simulink model "LukePractice"  (R2025a)
settings: Solver=VariableStepAuto  StartTime=0.0  StopTime=10.0  RelTol=1e-3
settings Model: Creator=jakeo  LastModifiedBy=lukef

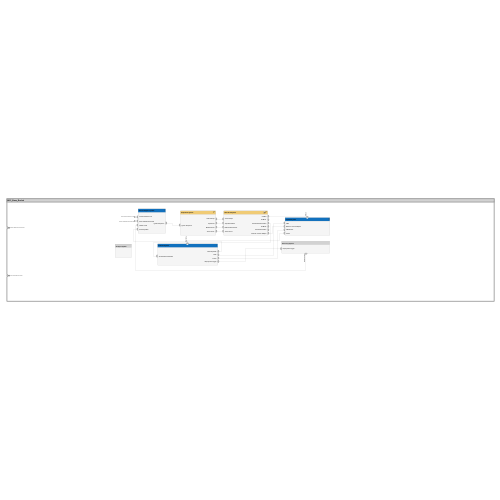
[thumbnail: Simulink's stored preview of the top-level diagram]
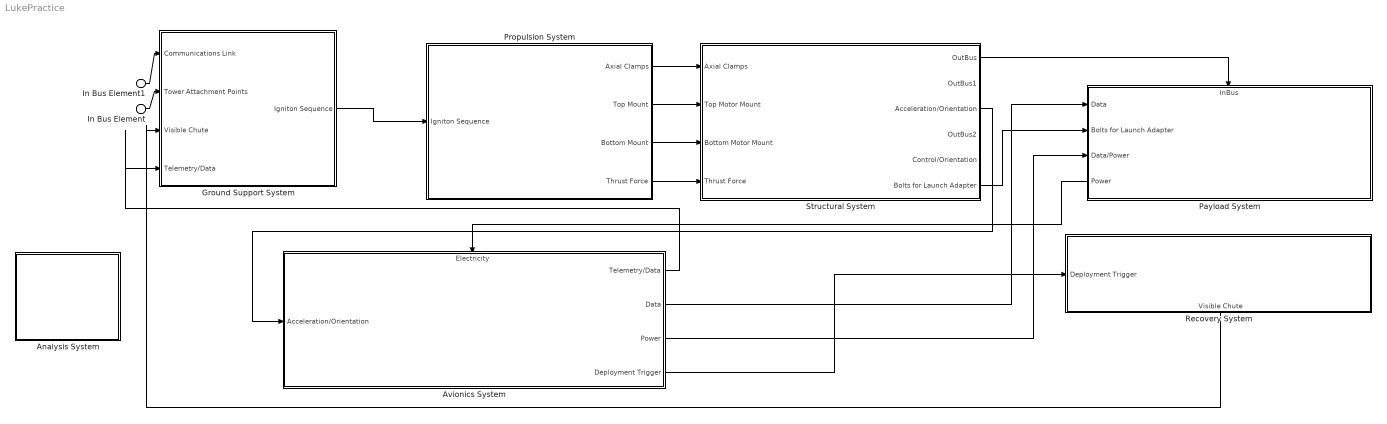
== system LukePractice ==
  In Bus Element : Inport  PortName=Tower Attachment Points
  In Bus Element1 : Inport  Port=2  PortName=Communications Link
  Analysis System : Subsystem
      settings: PortSchema="{\"entries\":[{\"content\":{\"headerSize\":26,\"margin\":15,\"minimumSpacing\":25,\"sides\":[{\"content\":{},\"type\":\"ConnectorPlacement.EquallySpacedRectSide\",\"uuid\":\"cc45333b-0876-4849-98d5-148de8a70f6b\"},{\"content\":{\"side\":\"RIGHT\"},\"type\":\"ConnectorPlacement.EquallySpacedRectSide\",\"uuid\":\"6d7662cc-0b93-4c22-b72a-22299e415e66\"},{\"content\":{\"side\":\"TOP\"},\"type\":\"ConnectorPlacement.EquallySpacedRectSide\",\"uuid\":\"98fed930-52bb-4e3d-bf56-50c036dee122\"}]},\"type\":\"ConnectorPlacement.EquallySpacedConnector\",\"uuid\":\"dfbe24ca-e965-4cbc-a32c-fe604c746b0d\"}],\"packageUris\":[\"http://schema.mathworks.com/mf0/Connector/R2020b\"],\"version\":\"1.0\"}"
  Avionics System : Subsystem
      settings: PortSchema="{\"entries\":[{\"content\":{\"headerSize\":26,\"margin\":15,\"minimumSpacing\":25,\"sides\":[{\"content\":{\"connectorIds\":[\"In2\"]},\"type\":\"ConnectorPlacement.EquallySpacedRectSide\",\"uuid\":\"6d56020f-32f3-4fce-baf0-a88f7155ace1\"},{\"content\":{\"connectorIds\":[\"Out1\",\"Out2\",\"Out3\",\"Out4\"],\"side\":\"RIGHT\"},\"type\":\"ConnectorPlacement.EquallySpacedRectSide\",\"uuid\":\"c9981725-d77c-44c3-a293-bb000501b1f7\"},{\"content\":{\"connectorIds\":[\"In1\"],\"side\":\"TOP\"},\"type\":\"ConnectorPlacement.EquallySpacedRectSide\",\"uuid\":\"9359d402-59c0-4829-a327-e8f675a7e108\"}]},\"type\":\"ConnectorPlacement.EquallySpacedConnector\",\"uuid\":\"22d4e63e-7f95-4c47-b029-dffe7490f4e3\"}],\"packageUris\":[\"http://schema.mathworks.com/mf0/Connector/R2020b\"],\"version\":\"1.0\"}"
  Ground Support System : Subsystem
      settings: PortSchema="{\"entries\":[{\"content\":{\"headerSize\":26,\"margin\":15,\"minimumSpacing\":25,\"sides\":[{\"content\":{\"connectorIds\":[\"In1\",\"In4\",\"In3\",\"In2\"]},\"type\":\"ConnectorPlacement.EquallySpacedRectSide\",\"uuid\":\"6d56020f-32f3-4fce-baf0-a88f7155ace1\"},{\"content\":{\"connectorIds\":[\"Out1\"],\"side\":\"RIGHT\"},\"type\":\"ConnectorPlacement.EquallySpacedRectSide\",\"uuid\":\"c9981725-d77c-44c3-a293-bb000501b1f7\"},{\"content\":{\"side\":\"TOP\"},\"type\":\"ConnectorPlacement.EquallySpacedRectSide\",\"uuid\":\"9359d402-59c0-4829-a327-e8f675a7e108\"},{\"content\":{\"side\":\"BOTTOM\"},\"type\":\"ConnectorPlacement.EquallySpacedRectSide\",\"uuid\":\"0562d536-5ab7-4f95-b231-de77c5a317a2\"}]},\"type\":\"ConnectorPlacement.EquallySpacedConnector\",\"uuid\":\"22d4e63e-7f95-4c47-b029-dffe7490f4e3\"}],\"packageUris\":[\"http://schema.mathworks.com/mf0/Connector/R2020b\"],\"version\":\"1.0\"}"
  Payload System : Subsystem
      settings: PortSchema="{\"entries\":[{\"content\":{\"headerSize\":26,\"margin\":15,\"minimumSpacing\":25,\"sides\":[{\"content\":{\"connectorIds\":[\"In1\",\"In2\",\"In4\",\"Out1\"]},\"type\":\"ConnectorPlacement.EquallySpacedRectSide\",\"uuid\":\"6d56020f-32f3-4fce-baf0-a88f7155ace1\"},{\"content\":{\"side\":\"RIGHT\"},\"type\":\"ConnectorPlacement.EquallySpacedRectSide\",\"uuid\":\"c9981725-d77c-44c3-a293-bb000501b1f7\"},{\"content\":{\"connectorIds\":[\"In3\"],\"side\":\"TOP\"},\"type\":\"ConnectorPlacement.EquallySpacedRectSide\",\"uuid\":\"9359d402-59c0-4829-a327-e8f675a7e108\"}]},\"type\":\"ConnectorPlacement.EquallySpacedConnector\",\"uuid\":\"22d4e63e-7f95-4c47-b029-dffe7490f4e3\"}],\"packageUris\":[\"http://schema.mathworks.com/mf0/Connector/R2020b\"],\"version\":\"1.0\"}"
  Propulsion System : Subsystem
      settings: PortSchema="{\"entries\":[{\"content\":{\"headerSize\":26,\"margin\":15,\"minimumSpacing\":25,\"sides\":[{\"content\":{\"connectorIds\":[\"In1\"]},\"type\":\"ConnectorPlacement.EquallySpacedRectSide\",\"uuid\":\"6d56020f-32f3-4fce-baf0-a88f7155ace1\"},{\"content\":{\"connectorIds\":[\"Out1\",\"Out2\",\"Out3\",\"Out4\"],\"side\":\"RIGHT\"},\"type\":\"ConnectorPlacement.EquallySpacedRectSide\",\"uuid\":\"c9981725-d77c-44c3-a293-bb000501b1f7\"},{\"content\":{\"side\":\"TOP\"},\"type\":\"ConnectorPlacement.EquallySpacedRectSide\",\"uuid\":\"9359d402-59c0-4829-a327-e8f675a7e108\"},{\"content\":{\"side\":\"BOTTOM\"},\"type\":\"ConnectorPlacement.EquallySpacedRectSide\",\"uuid\":\"2f60ee6a-ee89-41bf-8f54-e5ad8be751a0\"}]},\"type\":\"ConnectorPlacement.EquallySpacedConnector\",\"uuid\":\"22d4e63e-7f95-4c47-b029-dffe7490f4e3\"}],\"packageUris\":[\"http://schema.mathworks.com/mf0/Connector/R2020b\"],\"version\":\"1.0\"}"
  Recovery System : Subsystem
      settings: PortSchema="{\"entries\":[{\"content\":{\"headerSize\":26,\"margin\":15,\"minimumSpacing\":25,\"sides\":[{\"content\":{\"connectorIds\":[\"In1\"]},\"type\":\"ConnectorPlacement.EquallySpacedRectSide\",\"uuid\":\"6d56020f-32f3-4fce-baf0-a88f7155ace1\"},{\"content\":{\"side\":\"RIGHT\"},\"type\":\"ConnectorPlacement.EquallySpacedRectSide\",\"uuid\":\"c9981725-d77c-44c3-a293-bb000501b1f7\"},{\"content\":{\"side\":\"TOP\"},\"type\":\"ConnectorPlacement.EquallySpacedRectSide\",\"uuid\":\"9359d402-59c0-4829-a327-e8f675a7e108\"},{\"content\":{\"connectorIds\":[\"Out1\"],\"side\":\"BOTTOM\"},\"type\":\"ConnectorPlacement.EquallySpacedRectSide\",\"uuid\":\"84cb8274-0faa-44eb-ac5a-c7f9ad04c935\"}]},\"type\":\"ConnectorPlacement.EquallySpacedConnector\",\"uuid\":\"22d4e63e-7f95-4c47-b029-dffe7490f4e3\"}],\"packageUris\":[\"http://schema.mathworks.com/mf0/Connector/R2020b\"],\"version\":\"1.0\"}"
  Structural System : Subsystem
      settings: PortSchema="{\"entries\":[{\"content\":{\"headerSize\":26,\"margin\":15,\"minimumSpacing\":25,\"sides\":[{\"content\":{\"connectorIds\":[\"In1\",\"In2\",\"In3\",\"In4\"]},\"type\":\"ConnectorPlacement.EquallySpacedRectSide\",\"uuid\":\"6d56020f-32f3-4fce-baf0-a88f7155ace1\"},{\"content\":{\"connectorIds\":[\"Out1\",\"Out2\",\"Out3\",\"Out4\",\"Out5\",\"Out6\"],\"side\":\"RIGHT\"},\"type\":\"ConnectorPlacement.EquallySpacedRectSide\",\"uuid\":\"c9981725-d77c-44c3-a293-bb000501b1f7\"},{\"content\":{\"side\":\"TOP\"},\"type\":\"ConnectorPlacement.EquallySpacedRectSide\",\"uuid\":\"9359d402-59c0-4829-a327-e8f675a7e108\"}]},\"type\":\"ConnectorPlacement.EquallySpacedConnector\",\"uuid\":\"22d4e63e-7f95-4c47-b029-dffe7490f4e3\"}],\"packageUris\":[\"http://schema.mathworks.com/mf0/Connector/R2020b\"],\"version\":\"1.0\"}"
  wires:
  In Bus Element/1 -> Ground Support System/4(Tower Attachment Points)
  Propulsion System/4(Thrust Force) -> Structural System/4(Thrust Force)
  Avionics System/4(Deployment Trigger) -> Recovery System/1(Deployment Trigger)
  Avionics System/3(Power) -> Payload System/4(Data/Power)
  Avionics System/1(Telemetry/Data) -> Ground Support System/2(Telemetry/Data)
  Structural System/3(Acceleration/Orientation) -> Avionics System/2(Acceleration/Orientation)
  Ground Support System/1(Igniton Sequence) -> Propulsion System/1(Igniton Sequence)
  Structural System/1(OutBus) -> Payload System/3(InBus)
  Recovery System/1(Visible Chute) -> Ground Support System/3(Visible Chute)
  In Bus Element1/1 -> Ground Support System/1(Communications Link)
  Propulsion System/3(Bottom Mount) -> Structural System/3(Bottom Motor Mount)
  Propulsion System/2(Top Mount) -> Structural System/2(Top Motor Mount)
  Avionics System/2(Data) -> Payload System/1(Data)
  Payload System/1(Power) -> Avionics System/1(Electricity)
  Structural System/6(Bolts for Launch Adapter) -> Payload System/2(Bolts for Launch Adapter)
  Propulsion System/1(Axial Clamps) -> Structural System/1(Axial Clamps)

== system LukePractice/Analysis System ==

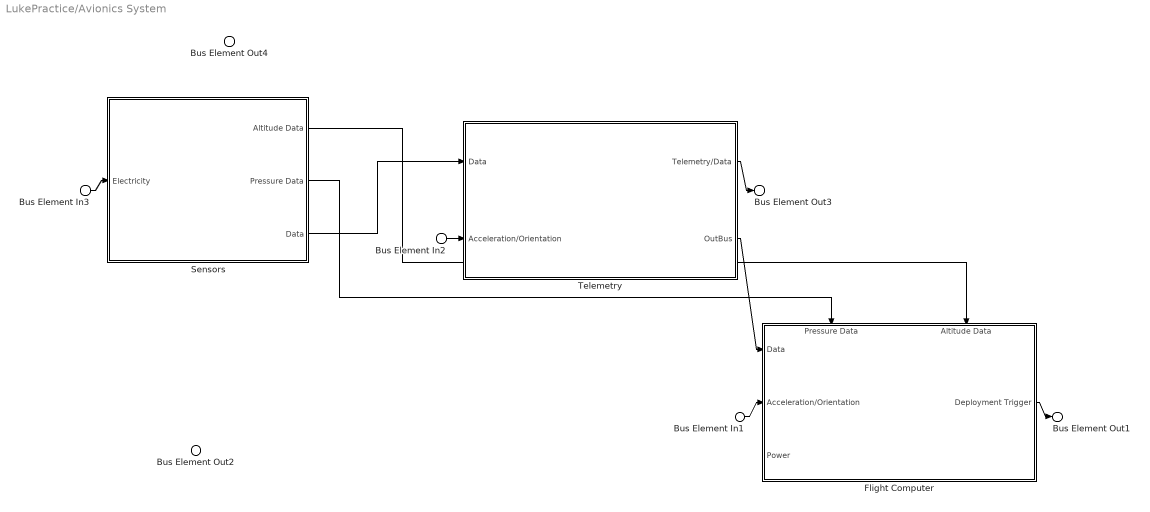
== system LukePractice/Avionics System ==
  Bus Element In3 : Inport  PortName=Electricity
  Bus Element In1 : Inport  Port=2  PortName=Acceleration/Orientation
  Bus Element In2 : Inport  Port=2  PortName=Acceleration/Orientation
  Flight Computer : Subsystem
      settings: PortSchema="{\"entries\":[{\"content\":{\"headerSize\":26,\"margin\":15,\"minimumSpacing\":25,\"sides\":[{\"content\":{\"connectorIds\":[\"In3\",\"In4\",\"In5\"]},\"type\":\"ConnectorPlacement.EquallySpacedRectSide\",\"uuid\":\"6d56020f-32f3-4fce-baf0-a88f7155ace1\"},{\"content\":{\"connectorIds\":[\"Out1\"],\"side\":\"RIGHT\"},\"type\":\"ConnectorPlacement.EquallySpacedRectSide\",\"uuid\":\"c9981725-d77c-44c3-a293-bb000501b1f7\"},{\"content\":{\"connectorIds\":[\"In1\",\"In2\"],\"side\":\"TOP\"},\"type\":\"ConnectorPlacement.EquallySpacedRectSide\",\"uuid\":\"9359d402-59c0-4829-a327-e8f675a7e108\"}]},\"type\":\"ConnectorPlacement.EquallySpacedConnector\",\"uuid\":\"22d4e63e-7f95-4c47-b029-dffe7490f4e3\"}],\"packageUris\":[\"http://schema.mathworks.com/mf0/Connector/R2020b\"],\"version\":\"1.0\"}"
  Sensors : Subsystem
      settings: PortSchema="{\"entries\":[{\"content\":{\"headerSize\":26,\"margin\":15,\"minimumSpacing\":25,\"sides\":[{\"content\":{\"connectorIds\":[\"In1\"]},\"type\":\"ConnectorPlacement.EquallySpacedRectSide\",\"uuid\":\"6d56020f-32f3-4fce-baf0-a88f7155ace1\"},{\"content\":{\"connectorIds\":[\"Out1\",\"Out2\",\"Out3\"],\"side\":\"RIGHT\"},\"type\":\"ConnectorPlacement.EquallySpacedRectSide\",\"uuid\":\"c9981725-d77c-44c3-a293-bb000501b1f7\"},{\"content\":{\"side\":\"TOP\"},\"type\":\"ConnectorPlacement.EquallySpacedRectSide\",\"uuid\":\"9359d402-59c0-4829-a327-e8f675a7e108\"}]},\"type\":\"ConnectorPlacement.EquallySpacedConnector\",\"uuid\":\"22d4e63e-7f95-4c47-b029-dffe7490f4e3\"}],\"packageUris\":[\"http://schema.mathworks.com/mf0/Connector/R2020b\"],\"version\":\"1.0\"}"
  Telemetry : Subsystem
      settings: PortSchema="{\"entries\":[{\"content\":{\"headerSize\":26,\"margin\":15,\"minimumSpacing\":25,\"sides\":[{\"content\":{\"connectorIds\":[\"In1\",\"In2\"]},\"type\":\"ConnectorPlacement.EquallySpacedRectSide\",\"uuid\":\"6d56020f-32f3-4fce-baf0-a88f7155ace1\"},{\"content\":{\"connectorIds\":[\"Out1\",\"Out2\"],\"side\":\"RIGHT\"},\"type\":\"ConnectorPlacement.EquallySpacedRectSide\",\"uuid\":\"c9981725-d77c-44c3-a293-bb000501b1f7\"},{\"content\":{\"side\":\"TOP\"},\"type\":\"ConnectorPlacement.EquallySpacedRectSide\",\"uuid\":\"9359d402-59c0-4829-a327-e8f675a7e108\"}]},\"type\":\"ConnectorPlacement.EquallySpacedConnector\",\"uuid\":\"22d4e63e-7f95-4c47-b029-dffe7490f4e3\"}],\"packageUris\":[\"http://schema.mathworks.com/mf0/Connector/R2020b\"],\"version\":\"1.0\"}"
  Bus Element Out3 : Outport  PortName=Telemetry/Data
  Bus Element Out4 : Outport  Port=2  PortName=Data
  Bus Element Out2 : Outport  Port=3  PortName=Power
  Bus Element Out1 : Outport  Port=4  PortName=Deployment Trigger
  wires:
  Bus Element In1/1 -> Flight Computer/4(Acceleration/Orientation)
  Sensors/3(Data) -> Telemetry/1(Data)
  Telemetry/2(OutBus) -> Flight Computer/3(Data)
  Bus Element In2/1 -> Telemetry/2(Acceleration/Orientation)
  Telemetry/1(Telemetry/Data) -> Bus Element Out3/1
  Flight Computer/1(Deployment Trigger) -> Bus Element Out1/1
  Sensors/2(Pressure Data) -> Flight Computer/1(Pressure Data)
  Sensors/1(Altitude Data) -> Flight Computer/2(Altitude Data)
  Bus Element In3/1 -> Sensors/1(Electricity)

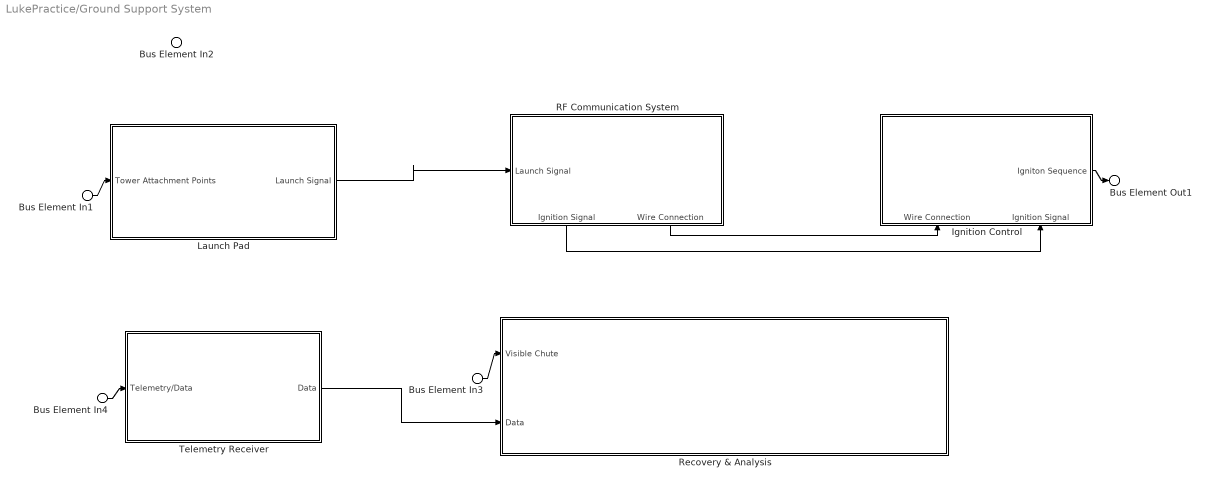
== system LukePractice/Ground Support System ==
  Bus Element In2 : Inport  PortName=Communications Link
  Bus Element In4 : Inport  Port=2  PortName=Telemetry/Data
  Bus Element In3 : Inport  Port=3  PortName=Visible Chute
  Bus Element In1 : Inport  Port=4  PortName=Tower Attachment Points
  Ignition Control : Subsystem
      settings: PortSchema="{\"entries\":[{\"content\":{\"headerSize\":26,\"margin\":15,\"minimumSpacing\":25,\"sides\":[{\"content\":{},\"type\":\"ConnectorPlacement.EquallySpacedRectSide\",\"uuid\":\"6d56020f-32f3-4fce-baf0-a88f7155ace1\"},{\"content\":{\"connectorIds\":[\"Out1\"],\"side\":\"RIGHT\"},\"type\":\"ConnectorPlacement.EquallySpacedRectSide\",\"uuid\":\"c9981725-d77c-44c3-a293-bb000501b1f7\"},{\"content\":{\"side\":\"TOP\"},\"type\":\"ConnectorPlacement.EquallySpacedRectSide\",\"uuid\":\"9359d402-59c0-4829-a327-e8f675a7e108\"},{\"content\":{\"connectorIds\":[\"In1\",\"In2\"],\"side\":\"BOTTOM\"},\"type\":\"ConnectorPlacement.EquallySpacedRectSide\",\"uuid\":\"b26f05fe-132d-4676-8ad1-7fecac435fa8\"}]},\"type\":\"ConnectorPlacement.EquallySpacedConnector\",\"uuid\":\"22d4e63e-7f95-4c47-b029-dffe7490f4e3\"}],\"packageUris\":[\"http://schema.mathworks.com/mf0/Connector/R2020b\"],\"version\":\"1.0\"}"
  Launch Pad : Subsystem
      settings: PortSchema="{\"entries\":[{\"content\":{\"headerSize\":26,\"margin\":15,\"minimumSpacing\":25,\"sides\":[{\"content\":{\"connectorIds\":[\"In1\"]},\"type\":\"ConnectorPlacement.EquallySpacedRectSide\",\"uuid\":\"6d56020f-32f3-4fce-baf0-a88f7155ace1\"},{\"content\":{\"connectorIds\":[\"Out1\"],\"side\":\"RIGHT\"},\"type\":\"ConnectorPlacement.EquallySpacedRectSide\",\"uuid\":\"c9981725-d77c-44c3-a293-bb000501b1f7\"},{\"content\":{\"side\":\"TOP\"},\"type\":\"ConnectorPlacement.EquallySpacedRectSide\",\"uuid\":\"9359d402-59c0-4829-a327-e8f675a7e108\"}]},\"type\":\"ConnectorPlacement.EquallySpacedConnector\",\"uuid\":\"22d4e63e-7f95-4c47-b029-dffe7490f4e3\"}],\"packageUris\":[\"http://schema.mathworks.com/mf0/Connector/R2020b\"],\"version\":\"1.0\"}"
  RF Communication System : Subsystem
      settings: PortSchema="{\"entries\":[{\"content\":{\"headerSize\":26,\"margin\":15,\"minimumSpacing\":25,\"sides\":[{\"content\":{\"connectorIds\":[\"In1\"]},\"type\":\"ConnectorPlacement.EquallySpacedRectSide\",\"uuid\":\"6d56020f-32f3-4fce-baf0-a88f7155ace1\"},{\"content\":{\"side\":\"RIGHT\"},\"type\":\"ConnectorPlacement.EquallySpacedRectSide\",\"uuid\":\"c9981725-d77c-44c3-a293-bb000501b1f7\"},{\"content\":{\"side\":\"TOP\"},\"type\":\"ConnectorPlacement.EquallySpacedRectSide\",\"uuid\":\"9359d402-59c0-4829-a327-e8f675a7e108\"},{\"content\":{\"connectorIds\":[\"Out1\",\"Out2\"],\"side\":\"BOTTOM\"},\"type\":\"ConnectorPlacement.EquallySpacedRectSide\",\"uuid\":\"ccd2d326-55bc-4419-a15b-a3180bff0ee7\"}]},\"type\":\"ConnectorPlacement.EquallySpacedConnector\",\"uuid\":\"22d4e63e-7f95-4c47-b029-dffe7490f4e3\"}],\"packageUris\":[\"http://schema.mathworks.com/mf0/Connector/R2020b\"],\"version\":\"1.0\"}"
  Recovery & Analysis : Subsystem
      settings: PortSchema="{\"entries\":[{\"content\":{\"headerSize\":26,\"margin\":15,\"minimumSpacing\":25,\"sides\":[{\"content\":{\"connectorIds\":[\"In1\",\"In2\"]},\"type\":\"ConnectorPlacement.EquallySpacedRectSide\",\"uuid\":\"2e13f5a1-d12d-4e78-8c7d-b3419191e00e\"},{\"content\":{\"side\":\"RIGHT\"},\"type\":\"ConnectorPlacement.EquallySpacedRectSide\",\"uuid\":\"2e54f79d-d26c-4f1e-aad7-d167a8605581\"},{\"content\":{\"side\":\"TOP\"},\"type\":\"ConnectorPlacement.EquallySpacedRectSide\",\"uuid\":\"127632d1-acf1-4856-b80a-47a4730bf8fe\"}]},\"type\":\"ConnectorPlacement.EquallySpacedConnector\",\"uuid\":\"7fb5950c-eb56-4ad7-bb81-f4b7b8097c7f\"}],\"packageUris\":[\"http://schema.mathworks.com/mf0/Connector/R2020b\"],\"version\":\"1.0\"}"
  Telemetry Receiver : Subsystem
      settings: PortSchema="{\"entries\":[{\"content\":{\"headerSize\":26,\"margin\":15,\"minimumSpacing\":25,\"sides\":[{\"content\":{\"connectorIds\":[\"In1\"]},\"type\":\"ConnectorPlacement.EquallySpacedRectSide\",\"uuid\":\"6d56020f-32f3-4fce-baf0-a88f7155ace1\"},{\"content\":{\"connectorIds\":[\"Out1\"],\"side\":\"RIGHT\"},\"type\":\"ConnectorPlacement.EquallySpacedRectSide\",\"uuid\":\"c9981725-d77c-44c3-a293-bb000501b1f7\"},{\"content\":{\"side\":\"TOP\"},\"type\":\"ConnectorPlacement.EquallySpacedRectSide\",\"uuid\":\"9359d402-59c0-4829-a327-e8f675a7e108\"}]},\"type\":\"ConnectorPlacement.EquallySpacedConnector\",\"uuid\":\"22d4e63e-7f95-4c47-b029-dffe7490f4e3\"}],\"packageUris\":[\"http://schema.mathworks.com/mf0/Connector/R2020b\"],\"version\":\"1.0\"}"
  Bus Element Out1 : Outport  PortName=Igniton Sequence
  wires:
  Bus Element In3/1 -> Recovery & Analysis/1(Visible Chute)
  Bus Element In1/1 -> Launch Pad/1(Tower Attachment Points)
  Bus Element In4/1 -> Telemetry Receiver/1(Telemetry/Data)
  Telemetry Receiver/1(Data) -> Recovery & Analysis/2(Data)
  Launch Pad/1(Launch Signal) -> RF Communication System/1(Launch Signal)
  RF Communication System/1(Ignition Signal) -> Ignition Control/2(Ignition Signal)
  Ignition Control/1(Igniton Sequence) -> Bus Element Out1/1
  RF Communication System/2(Wire Connection) -> Ignition Control/1(Wire Connection)

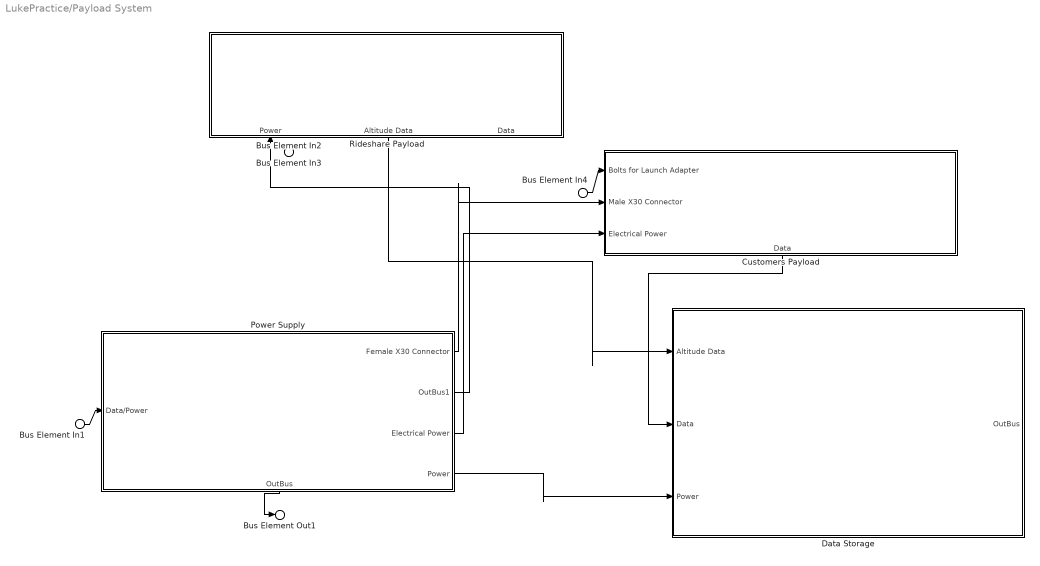
== system LukePractice/Payload System ==
  Bus Element In3 : Inport  PortName=Data
  Bus Element In4 : Inport  Port=2  PortName=Bolts for Launch Adapter
  Bus Element In2 : Inport  Port=3  PortName=InBus
  Bus Element In1 : Inport  Port=4  PortName=Data/Power
  Customers Payload : Subsystem
      settings: PortSchema="{\"entries\":[{\"content\":{\"headerSize\":26,\"margin\":15,\"minimumSpacing\":25,\"sides\":[{\"content\":{\"connectorIds\":[\"In1\",\"In2\",\"In3\"]},\"type\":\"ConnectorPlacement.EquallySpacedRectSide\",\"uuid\":\"6d56020f-32f3-4fce-baf0-a88f7155ace1\"},{\"content\":{\"side\":\"RIGHT\"},\"type\":\"ConnectorPlacement.EquallySpacedRectSide\",\"uuid\":\"c9981725-d77c-44c3-a293-bb000501b1f7\"},{\"content\":{\"side\":\"TOP\"},\"type\":\"ConnectorPlacement.EquallySpacedRectSide\",\"uuid\":\"9359d402-59c0-4829-a327-e8f675a7e108\"},{\"content\":{\"connectorIds\":[\"Out1\"],\"side\":\"BOTTOM\"},\"type\":\"ConnectorPlacement.EquallySpacedRectSide\",\"uuid\":\"17812ff1-462a-44f7-abf9-931c8845ebf9\"}]},\"type\":\"ConnectorPlacement.EquallySpacedConnector\",\"uuid\":\"22d4e63e-7f95-4c47-b029-dffe7490f4e3\"}],\"packageUris\":[\"http://schema.mathworks.com/mf0/Connector/R2020b\"],\"version\":\"1.0\"}"
  Data Storage : Subsystem
      settings: PortSchema="{\"entries\":[{\"content\":{\"headerSize\":26,\"margin\":15,\"minimumSpacing\":25,\"sides\":[{\"content\":{\"connectorIds\":[\"In1\",\"In2\",\"In3\"]},\"type\":\"ConnectorPlacement.EquallySpacedRectSide\",\"uuid\":\"6d56020f-32f3-4fce-baf0-a88f7155ace1\"},{\"content\":{\"connectorIds\":[\"Out1\"],\"side\":\"RIGHT\"},\"type\":\"ConnectorPlacement.EquallySpacedRectSide\",\"uuid\":\"c9981725-d77c-44c3-a293-bb000501b1f7\"},{\"content\":{\"side\":\"TOP\"},\"type\":\"ConnectorPlacement.EquallySpacedRectSide\",\"uuid\":\"9359d402-59c0-4829-a327-e8f675a7e108\"}]},\"type\":\"ConnectorPlacement.EquallySpacedConnector\",\"uuid\":\"22d4e63e-7f95-4c47-b029-dffe7490f4e3\"}],\"packageUris\":[\"http://schema.mathworks.com/mf0/Connector/R2020b\"],\"version\":\"1.0\"}"
  "Power Supply " : Subsystem
      settings: PortSchema="{\"entries\":[{\"content\":{\"headerSize\":26,\"margin\":15,\"minimumSpacing\":25,\"sides\":[{\"content\":{\"connectorIds\":[\"In1\"]},\"type\":\"ConnectorPlacement.EquallySpacedRectSide\",\"uuid\":\"6d56020f-32f3-4fce-baf0-a88f7155ace1\"},{\"content\":{\"connectorIds\":[\"Out1\",\"Out3\",\"Out4\",\"Out5\"],\"side\":\"RIGHT\"},\"type\":\"ConnectorPlacement.EquallySpacedRectSide\",\"uuid\":\"c9981725-d77c-44c3-a293-bb000501b1f7\"},{\"content\":{\"side\":\"TOP\"},\"type\":\"ConnectorPlacement.EquallySpacedRectSide\",\"uuid\":\"9359d402-59c0-4829-a327-e8f675a7e108\"},{\"content\":{\"connectorIds\":[\"Out2\"],\"side\":\"BOTTOM\"},\"type\":\"ConnectorPlacement.EquallySpacedRectSide\",\"uuid\":\"3de9e842-ce67-4c70-8973-3088f80d4735\"}]},\"type\":\"ConnectorPlacement.EquallySpacedConnector\",\"uuid\":\"22d4e63e-7f95-4c47-b029-dffe7490f4e3\"}],\"packageUris\":[\"http://schema.mathworks.com/mf0/Connector/R2020b\"],\"version\":\"1.0\"}"
  Rideshare Payload : Subsystem
      settings: PortSchema="{\"entries\":[{\"content\":{\"headerSize\":26,\"margin\":15,\"minimumSpacing\":25,\"sides\":[{\"content\":{},\"type\":\"ConnectorPlacement.EquallySpacedRectSide\",\"uuid\":\"2e13f5a1-d12d-4e78-8c7d-b3419191e00e\"},{\"content\":{\"side\":\"RIGHT\"},\"type\":\"ConnectorPlacement.EquallySpacedRectSide\",\"uuid\":\"2e54f79d-d26c-4f1e-aad7-d167a8605581\"},{\"content\":{\"side\":\"TOP\"},\"type\":\"ConnectorPlacement.EquallySpacedRectSide\",\"uuid\":\"127632d1-acf1-4856-b80a-47a4730bf8fe\"},{\"content\":{\"connectorIds\":[\"In1\",\"Out1\",\"Out2\"],\"side\":\"BOTTOM\"},\"type\":\"ConnectorPlacement.EquallySpacedRectSide\",\"uuid\":\"c99d9fe7-93a0-4b59-beae-ff6ce6a4fb80\"}]},\"type\":\"ConnectorPlacement.EquallySpacedConnector\",\"uuid\":\"7fb5950c-eb56-4ad7-bb81-f4b7b8097c7f\"}],\"packageUris\":[\"http://schema.mathworks.com/mf0/Connector/R2020b\"],\"version\":\"1.0\"}"
  Bus Element Out1 : Outport  PortName=Power
  wires:
  Bus Element In1/1 -> "Power Supply "/1(Data/Power)
  "Power Supply "/5(Power) -> Data Storage/3(Power)
  "Power Supply "/4(Electrical Power) -> Customers Payload/3(Electrical Power)
  Customers Payload/1(Data) -> Data Storage/2(Data)
  "Power Supply "/3(OutBus1) -> Rideshare Payload/1(Power)
  Rideshare Payload/1(Altitude Data) -> Data Storage/1(Altitude Data)
  "Power Supply "/2(OutBus) -> Bus Element Out1/1
  "Power Supply "/1(Female X30 Connector) -> Customers Payload/2(Male X30 Connector)
  Bus Element In4/1 -> Customers Payload/1(Bolts for Launch Adapter)

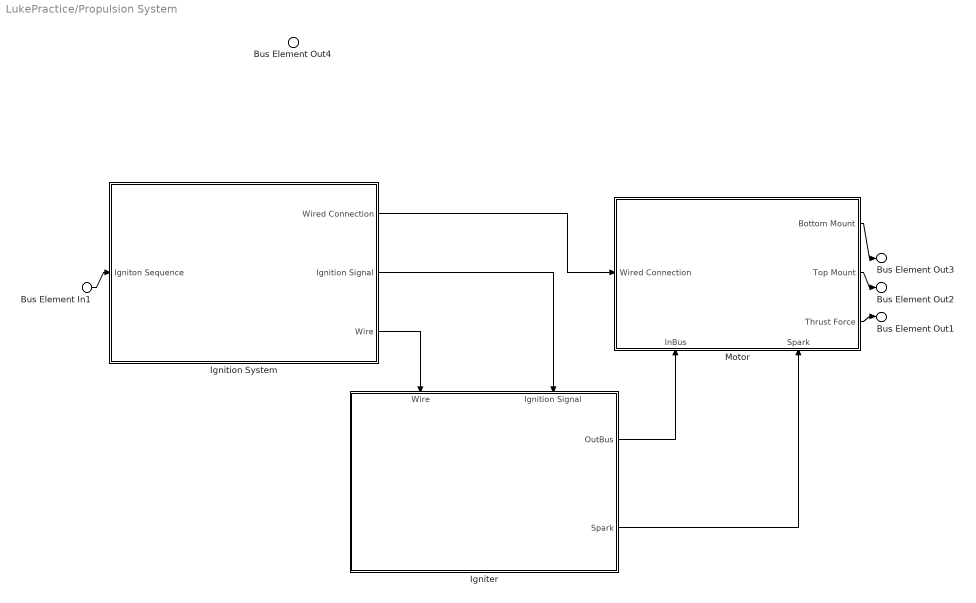
== system LukePractice/Propulsion System ==
  Bus Element In1 : Inport  PortName=Igniton Sequence
  Igniter : Subsystem
      settings: PortSchema="{\"entries\":[{\"content\":{\"headerSize\":26,\"margin\":15,\"minimumSpacing\":25,\"sides\":[{\"content\":{},\"type\":\"ConnectorPlacement.EquallySpacedRectSide\",\"uuid\":\"ee90fd67-ce3c-463a-922d-00379c91d92f\"},{\"content\":{\"connectorIds\":[\"Out1\",\"Out2\"],\"side\":\"RIGHT\"},\"type\":\"ConnectorPlacement.EquallySpacedRectSide\",\"uuid\":\"57bdd80c-9026-4844-a97e-bdf46341acf9\"},{\"content\":{\"connectorIds\":[\"In1\",\"In2\"],\"side\":\"TOP\"},\"type\":\"ConnectorPlacement.EquallySpacedRectSide\",\"uuid\":\"7c374427-6658-48c0-ad54-d8c414c813ef\"}]},\"type\":\"ConnectorPlacement.EquallySpacedConnector\",\"uuid\":\"baeb2d3f-30b1-4010-b9ee-d30a650b13c4\"}],\"packageUris\":[\"http://schema.mathworks.com/mf0/Connector/R2020b\"],\"version\":\"1.0\"}"
  Ignition System : Subsystem
      settings: PortSchema="{\"entries\":[{\"content\":{\"headerSize\":26,\"margin\":15,\"minimumSpacing\":25,\"sides\":[{\"content\":{\"connectorIds\":[\"In1\"]},\"type\":\"ConnectorPlacement.EquallySpacedRectSide\",\"uuid\":\"6d56020f-32f3-4fce-baf0-a88f7155ace1\"},{\"content\":{\"connectorIds\":[\"Out1\",\"Out2\",\"Out3\"],\"side\":\"RIGHT\"},\"type\":\"ConnectorPlacement.EquallySpacedRectSide\",\"uuid\":\"c9981725-d77c-44c3-a293-bb000501b1f7\"},{\"content\":{\"side\":\"TOP\"},\"type\":\"ConnectorPlacement.EquallySpacedRectSide\",\"uuid\":\"9359d402-59c0-4829-a327-e8f675a7e108\"}]},\"type\":\"ConnectorPlacement.EquallySpacedConnector\",\"uuid\":\"22d4e63e-7f95-4c47-b029-dffe7490f4e3\"}],\"packageUris\":[\"http://schema.mathworks.com/mf0/Connector/R2020b\"],\"version\":\"1.0\"}"
  "Motor " : Subsystem
      settings: PortSchema="{\"entries\":[{\"content\":{\"headerSize\":26,\"margin\":15,\"minimumSpacing\":25,\"sides\":[{\"content\":{\"connectorIds\":[\"In3\"]},\"type\":\"ConnectorPlacement.EquallySpacedRectSide\",\"uuid\":\"6d56020f-32f3-4fce-baf0-a88f7155ace1\"},{\"content\":{\"connectorIds\":[\"Out1\",\"Out2\",\"Out3\"],\"side\":\"RIGHT\"},\"type\":\"ConnectorPlacement.EquallySpacedRectSide\",\"uuid\":\"c9981725-d77c-44c3-a293-bb000501b1f7\"},{\"content\":{\"side\":\"TOP\"},\"type\":\"ConnectorPlacement.EquallySpacedRectSide\",\"uuid\":\"9359d402-59c0-4829-a327-e8f675a7e108\"},{\"content\":{\"connectorIds\":[\"In1\",\"In2\"],\"side\":\"BOTTOM\"},\"type\":\"ConnectorPlacement.EquallySpacedRectSide\",\"uuid\":\"11bdd568-2fef-4c3d-872d-f25645e90a0c\"}]},\"type\":\"ConnectorPlacement.EquallySpacedConnector\",\"uuid\":\"22d4e63e-7f95-4c47-b029-dffe7490f4e3\"}],\"packageUris\":[\"http://schema.mathworks.com/mf0/Connector/R2020b\"],\"version\":\"1.0\"}"
  Bus Element Out4 : Outport  PortName=Axial Clamps
  Bus Element Out2 : Outport  Port=2  PortName=Top Mount
  Bus Element Out3 : Outport  Port=3  PortName=Bottom Mount
  Bus Element Out1 : Outport  Port=4  PortName=Thrust Force
  wires:
  Bus Element In1/1 -> Ignition System/1(Igniton Sequence)
  "Motor "/3(Thrust Force) -> Bus Element Out1/1
  Ignition System/1(Wired Connection) -> "Motor "/3(Wired Connection)
  "Motor "/2(Top Mount) -> Bus Element Out2/1
  "Motor "/1(Bottom Mount) -> Bus Element Out3/1
  Ignition System/3(Wire) -> Igniter/1(Wire)
  Igniter/2(Spark) -> "Motor "/2(Spark)
  Ignition System/2(Ignition Signal) -> Igniter/2(" Ignition Signal")
  Igniter/1(OutBus) -> "Motor "/1(InBus)

== system LukePractice/Recovery System ==
  Bus Element In1 : Inport  PortName=Deployment Trigger
  Drogue Chute : Subsystem
      settings: PortSchema="{\"entries\":[{\"content\":{\"headerSize\":26,\"margin\":15,\"minimumSpacing\":25,\"sides\":[{\"content\":{\"connectorIds\":[\"In1\"]},\"type\":\"ConnectorPlacement.EquallySpacedRectSide\",\"uuid\":\"6d56020f-32f3-4fce-baf0-a88f7155ace1\"},{\"content\":{\"connectorIds\":[\"Out1\"],\"side\":\"RIGHT\"},\"type\":\"ConnectorPlacement.EquallySpacedRectSide\",\"uuid\":\"c9981725-d77c-44c3-a293-bb000501b1f7\"},{\"content\":{\"side\":\"TOP\"},\"type\":\"ConnectorPlacement.EquallySpacedRectSide\",\"uuid\":\"9359d402-59c0-4829-a327-e8f675a7e108\"}]},\"type\":\"ConnectorPlacement.EquallySpacedConnector\",\"uuid\":\"22d4e63e-7f95-4c47-b029-dffe7490f4e3\"}],\"packageUris\":[\"http://schema.mathworks.com/mf0/Connector/R2020b\"],\"version\":\"1.0\"}"
  Main Chute : Subsystem
      settings: PortSchema="{\"entries\":[{\"content\":{\"headerSize\":26,\"margin\":15,\"minimumSpacing\":25,\"sides\":[{\"content\":{\"connectorIds\":[\"In1\"]},\"type\":\"ConnectorPlacement.EquallySpacedRectSide\",\"uuid\":\"6d56020f-32f3-4fce-baf0-a88f7155ace1\"},{\"content\":{\"side\":\"RIGHT\"},\"type\":\"ConnectorPlacement.EquallySpacedRectSide\",\"uuid\":\"c9981725-d77c-44c3-a293-bb000501b1f7\"},{\"content\":{\"side\":\"TOP\"},\"type\":\"ConnectorPlacement.EquallySpacedRectSide\",\"uuid\":\"9359d402-59c0-4829-a327-e8f675a7e108\"},{\"content\":{\"connectorIds\":[\"Out1\"],\"side\":\"BOTTOM\"},\"type\":\"ConnectorPlacement.EquallySpacedRectSide\",\"uuid\":\"f809839c-bd2a-4c61-a037-fd3459666388\"}]},\"type\":\"ConnectorPlacement.EquallySpacedConnector\",\"uuid\":\"22d4e63e-7f95-4c47-b029-dffe7490f4e3\"}],\"packageUris\":[\"http://schema.mathworks.com/mf0/Connector/R2020b\"],\"version\":\"1.0\"}"
  Bus Element Out1 : Outport  PortName=Visible Chute
  wires:
  Bus Element In1/1 -> Drogue Chute/1(Deployment Trigger)
  Drogue Chute/1(OutBus) -> Main Chute/1(InBus)
  Main Chute/1(Visible Chute) -> Bus Element Out1/1

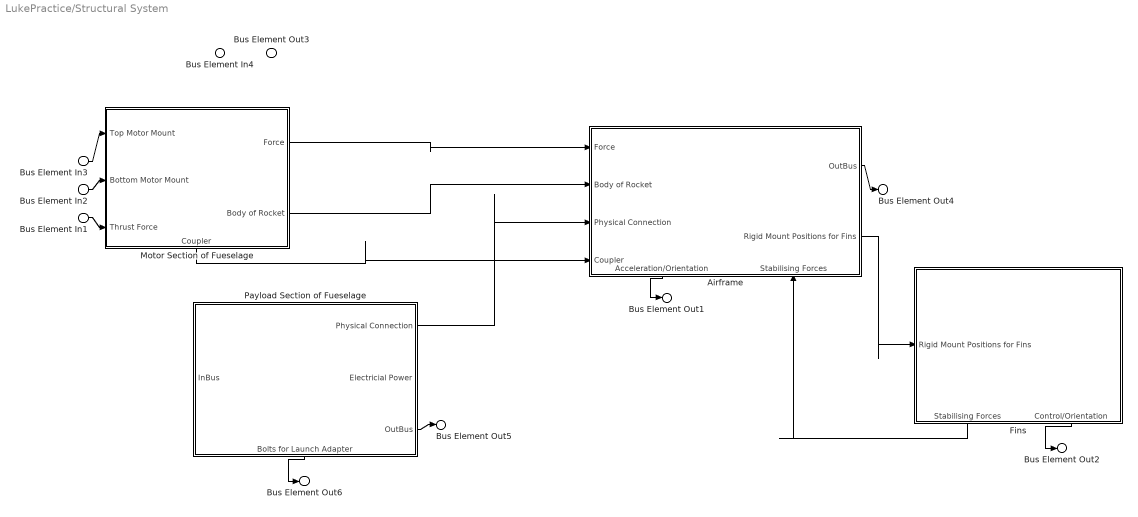
== system LukePractice/Structural System ==
  Bus Element In4 : Inport  PortName=Axial Clamps
  Bus Element In3 : Inport  Port=2  PortName=Top Motor Mount
  Bus Element In2 : Inport  Port=3  PortName=Bottom Motor Mount
  Bus Element In1 : Inport  Port=4  PortName=Thrust Force
  Airframe : Subsystem
      settings: PortSchema="{\"entries\":[{\"content\":{\"headerSize\":26,\"margin\":15,\"minimumSpacing\":25,\"sides\":[{\"content\":{\"connectorIds\":[\"In2\",\"In5\",\"In3\",\"In4\"]},\"type\":\"ConnectorPlacement.EquallySpacedRectSide\",\"uuid\":\"6d56020f-32f3-4fce-baf0-a88f7155ace1\"},{\"content\":{\"connectorIds\":[\"Out1\",\"Out3\"],\"side\":\"RIGHT\"},\"type\":\"ConnectorPlacement.EquallySpacedRectSide\",\"uuid\":\"c9981725-d77c-44c3-a293-bb000501b1f7\"},{\"content\":{\"side\":\"TOP\"},\"type\":\"ConnectorPlacement.EquallySpacedRectSide\",\"uuid\":\"9359d402-59c0-4829-a327-e8f675a7e108\"},{\"content\":{\"connectorIds\":[\"Out2\",\"In1\"],\"side\":\"BOTTOM\"},\"type\":\"ConnectorPlacement.EquallySpacedRectSide\",\"uuid\":\"1e7e0694-c431-49bf-9519-4fa148c41ab4\"}]},\"type\":\"ConnectorPlacement.EquallySpacedConnector\",\"uuid\":\"22d4e63e-7f95-4c47-b029-dffe7490f4e3\"}],\"packageUris\":[\"http://schema.mathworks.com/mf0/Connector/R2020b\"],\"version\":\"1.0\"}"
  Fins : Subsystem
      settings: PortSchema="{\"entries\":[{\"content\":{\"headerSize\":26,\"margin\":15,\"minimumSpacing\":25,\"sides\":[{\"content\":{\"connectorIds\":[\"In1\"]},\"type\":\"ConnectorPlacement.EquallySpacedRectSide\",\"uuid\":\"6d56020f-32f3-4fce-baf0-a88f7155ace1\"},{\"content\":{\"side\":\"RIGHT\"},\"type\":\"ConnectorPlacement.EquallySpacedRectSide\",\"uuid\":\"c9981725-d77c-44c3-a293-bb000501b1f7\"},{\"content\":{\"side\":\"TOP\"},\"type\":\"ConnectorPlacement.EquallySpacedRectSide\",\"uuid\":\"9359d402-59c0-4829-a327-e8f675a7e108\"},{\"content\":{\"connectorIds\":[\"Out1\",\"Out2\"],\"side\":\"BOTTOM\"},\"type\":\"ConnectorPlacement.EquallySpacedRectSide\",\"uuid\":\"934d0f44-d9ca-45cf-ac41-f0da4384728e\"}]},\"type\":\"ConnectorPlacement.EquallySpacedConnector\",\"uuid\":\"22d4e63e-7f95-4c47-b029-dffe7490f4e3\"}],\"packageUris\":[\"http://schema.mathworks.com/mf0/Connector/R2020b\"],\"version\":\"1.0\"}"
  Motor Section of Fueselage : Subsystem
      settings: PortSchema="{\"entries\":[{\"content\":{\"headerSize\":26,\"margin\":15,\"minimumSpacing\":25,\"sides\":[{\"content\":{\"connectorIds\":[\"In1\",\"In2\",\"In3\"]},\"type\":\"ConnectorPlacement.EquallySpacedRectSide\",\"uuid\":\"6d56020f-32f3-4fce-baf0-a88f7155ace1\"},{\"content\":{\"connectorIds\":[\"Out2\",\"Out3\"],\"side\":\"RIGHT\"},\"type\":\"ConnectorPlacement.EquallySpacedRectSide\",\"uuid\":\"c9981725-d77c-44c3-a293-bb000501b1f7\"},{\"content\":{\"side\":\"TOP\"},\"type\":\"ConnectorPlacement.EquallySpacedRectSide\",\"uuid\":\"9359d402-59c0-4829-a327-e8f675a7e108\"},{\"content\":{\"connectorIds\":[\"Out1\"],\"side\":\"BOTTOM\"},\"type\":\"ConnectorPlacement.EquallySpacedRectSide\",\"uuid\":\"dc71aef8-8f4a-4029-affd-9d9a45eb93ba\"}]},\"type\":\"ConnectorPlacement.EquallySpacedConnector\",\"uuid\":\"22d4e63e-7f95-4c47-b029-dffe7490f4e3\"}],\"packageUris\":[\"http://schema.mathworks.com/mf0/Connector/R2020b\"],\"version\":\"1.0\"}"
  Payload Section of Fueselage : Subsystem
      settings: PortSchema="{\"entries\":[{\"content\":{\"headerSize\":26,\"margin\":15,\"minimumSpacing\":25,\"sides\":[{\"content\":{\"connectorIds\":[\"In1\"]},\"type\":\"ConnectorPlacement.EquallySpacedRectSide\",\"uuid\":\"ee90fd67-ce3c-463a-922d-00379c91d92f\"},{\"content\":{\"connectorIds\":[\"Out2\",\"Out3\",\"Out4\"],\"side\":\"RIGHT\"},\"type\":\"ConnectorPlacement.EquallySpacedRectSide\",\"uuid\":\"57bdd80c-9026-4844-a97e-bdf46341acf9\"},{\"content\":{\"side\":\"TOP\"},\"type\":\"ConnectorPlacement.EquallySpacedRectSide\",\"uuid\":\"7c374427-6658-48c0-ad54-d8c414c813ef\"},{\"content\":{\"connectorIds\":[\"Out1\"],\"side\":\"BOTTOM\"},\"type\":\"ConnectorPlacement.EquallySpacedRectSide\",\"uuid\":\"ca12bc27-7abe-4ee5-9cb7-d693368c1440\"}]},\"type\":\"ConnectorPlacement.EquallySpacedConnector\",\"uuid\":\"baeb2d3f-30b1-4010-b9ee-d30a650b13c4\"}],\"packageUris\":[\"http://schema.mathworks.com/mf0/Connector/R2020b\"],\"version\":\"1.0\"}"
  Bus Element Out3 : Outport  PortName=OutBus
  Bus Element Out4 : Outport  Port=2  PortName=OutBus1
  Bus Element Out1 : Outport  Port=3  PortName=Acceleration/Orientation
  Bus Element Out5 : Outport  Port=4  PortName=OutBus2
  Bus Element Out2 : Outport  Port=5  PortName=Control/Orientation
  Bus Element Out6 : Outport  Port=6  PortName=Bolts for Launch Adapter
  wires:
  Bus Element In1/1 -> Motor Section of Fueselage/3(Thrust Force)
  Motor Section of Fueselage/2(Force) -> Airframe/2(Force)
  Airframe/3(Rigid Mount Positions for Fins) -> Fins/1(Rigid Mount Positions for Fins)
  Airframe/2(Acceleration/Orientation) -> Bus Element Out1/1
  Fins/2(Control/Orientation) -> Bus Element Out2/1
  Bus Element In3/1 -> Motor Section of Fueselage/1(Top Motor Mount)
  Bus Element In2/1 -> Motor Section of Fueselage/2(Bottom Motor Mount)
  Motor Section of Fueselage/3(Body of Rocket) -> Airframe/5(Body of Rocket)
  Fins/1(Stabilising Forces) -> Airframe/1(Stabilising Forces)
  Airframe/1(OutBus) -> Bus Element Out4/1
  Payload Section of Fueselage/2(Physical Connection) -> Airframe/3(Physical Connection)
  Payload Section of Fueselage/4(OutBus) -> Bus Element Out5/1
  Payload Section of Fueselage/1(Bolts for Launch Adapter) -> Bus Element Out6/1
  Motor Section of Fueselage/1("Coupler ") -> Airframe/4("Coupler ")

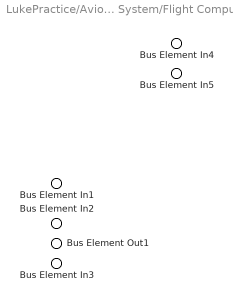
== system LukePractice/Avionics System/Flight Computer ==
  Bus Element In4 : Inport  PortName=Pressure Data
  Bus Element In5 : Inport  Port=2  PortName=Altitude Data
  Bus Element In1 : Inport  Port=3  PortName=Data
  Bus Element In2 : Inport  Port=4  PortName=Acceleration/Orientation
  Bus Element In3 : Inport  Port=5  PortName=Power
  Bus Element Out1 : Outport  PortName=Deployment Trigger

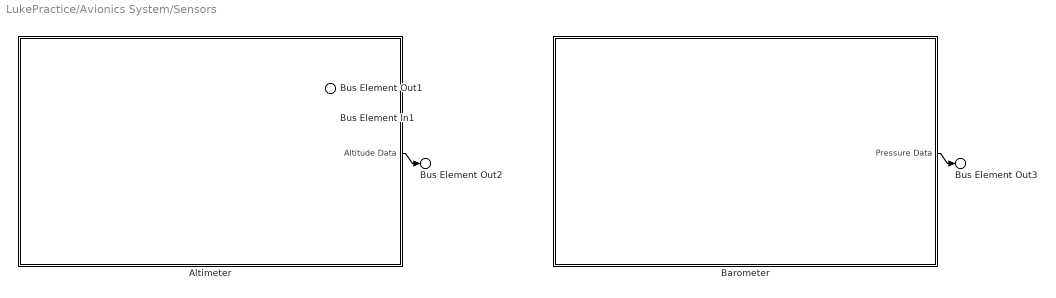
== system LukePractice/Avionics System/Sensors ==
  Bus Element In1 : Inport  PortName=Electricity
  Altimeter : Subsystem
      settings: PortSchema="{\"entries\":[{\"content\":{\"headerSize\":26,\"margin\":15,\"minimumSpacing\":25,\"sides\":[{\"content\":{},\"type\":\"ConnectorPlacement.EquallySpacedRectSide\",\"uuid\":\"ee90fd67-ce3c-463a-922d-00379c91d92f\"},{\"content\":{\"connectorIds\":[\"Out1\"],\"side\":\"RIGHT\"},\"type\":\"ConnectorPlacement.EquallySpacedRectSide\",\"uuid\":\"57bdd80c-9026-4844-a97e-bdf46341acf9\"},{\"content\":{\"side\":\"TOP\"},\"type\":\"ConnectorPlacement.EquallySpacedRectSide\",\"uuid\":\"7c374427-6658-48c0-ad54-d8c414c813ef\"}]},\"type\":\"ConnectorPlacement.EquallySpacedConnector\",\"uuid\":\"baeb2d3f-30b1-4010-b9ee-d30a650b13c4\"}],\"packageUris\":[\"http://schema.mathworks.com/mf0/Connector/R2020b\"],\"version\":\"1.0\"}"
  Barometer : Subsystem
      settings: PortSchema="{\"entries\":[{\"content\":{\"headerSize\":26,\"margin\":15,\"minimumSpacing\":25,\"sides\":[{\"content\":{},\"type\":\"ConnectorPlacement.EquallySpacedRectSide\",\"uuid\":\"ee90fd67-ce3c-463a-922d-00379c91d92f\"},{\"content\":{\"connectorIds\":[\"Out1\"],\"side\":\"RIGHT\"},\"type\":\"ConnectorPlacement.EquallySpacedRectSide\",\"uuid\":\"57bdd80c-9026-4844-a97e-bdf46341acf9\"},{\"content\":{\"side\":\"TOP\"},\"type\":\"ConnectorPlacement.EquallySpacedRectSide\",\"uuid\":\"7c374427-6658-48c0-ad54-d8c414c813ef\"}]},\"type\":\"ConnectorPlacement.EquallySpacedConnector\",\"uuid\":\"baeb2d3f-30b1-4010-b9ee-d30a650b13c4\"}],\"packageUris\":[\"http://schema.mathworks.com/mf0/Connector/R2020b\"],\"version\":\"1.0\"}"
  Bus Element Out2 : Outport  PortName=Altitude Data
  Bus Element Out3 : Outport  Port=2  PortName=Pressure Data
  Bus Element Out1 : Outport  Port=3  PortName=Data
  wires:
  Altimeter/1(Altitude Data) -> Bus Element Out2/1
  Barometer/1(Pressure Data) -> Bus Element Out3/1

== system LukePractice/Avionics System/Telemetry ==
  Bus Element In1 : Inport  PortName=Data
  Bus Element In2 : Inport  Port=2  PortName=Acceleration/Orientation
  Bus Element Out2 : Outport  PortName=Telemetry/Data
  Bus Element Out1 : Outport  Port=2  PortName=OutBus

== system LukePractice/Ground Support System/Ignition Control ==
  Bus Element In1 : Inport  PortName=Wire Connection
  Bus Element In2 : Inport  Port=2  PortName=Ignition Signal
  Bus Element Out1 : Outport  PortName=Igniton Sequence

== system LukePractice/Ground Support System/Launch Pad ==
  Bus Element In1 : Inport  PortName=Tower Attachment Points
  Bus Element Out2 : Outport  PortName=Launch Signal

== system LukePractice/Ground Support System/RF Communication System ==
  Bus Element In1 : Inport  PortName=Launch Signal
  Bus Element Out1 : Outport  PortName=Ignition Signal
  Bus Element Out2 : Outport  Port=2  PortName=Wire Connection

== system LukePractice/Ground Support System/Recovery & Analysis ==
  Bus Element In2 : Inport  PortName=Visible Chute
  Bus Element In1 : Inport  Port=2  PortName=Data

== system LukePractice/Ground Support System/Telemetry Receiver ==
  Bus Element In1 : Inport  PortName=Telemetry/Data
  Bus Element Out1 : Outport  PortName=Data

== system LukePractice/Payload System/Customers Payload ==
  Bus Element In3 : Inport  PortName=Bolts for Launch Adapter
  Bus Element In2 : Inport  Port=2  PortName=Male X30 Connector
  Bus Element In1 : Inport  Port=3  PortName=Electrical Power
  Bus Element Out1 : Outport  PortName=Data

== system LukePractice/Payload System/Data Storage ==
  Bus Element In3 : Inport  PortName=Altitude Data
  Bus Element In2 : Inport  Port=2  PortName=Data
  Bus Element In1 : Inport  Port=3  PortName=Power
  Bus Element Out1 : Outport  PortName=OutBus

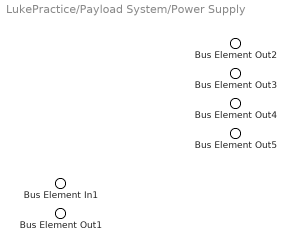
== system LukePractice/Payload System/Power Supply  ==
  Bus Element In1 : Inport  PortName=Data/Power
  Bus Element Out5 : Outport  PortName=Female X30 Connector
  Bus Element Out4 : Outport  Port=2  PortName=OutBus
  Bus Element Out3 : Outport  Port=3  PortName=OutBus1
  Bus Element Out2 : Outport  Port=4  PortName=Electrical Power
  Bus Element Out1 : Outport  Port=5  PortName=Power

== system LukePractice/Payload System/Rideshare Payload ==
  Bus Element In1 : Inport  PortName=Power
  Altimeter : Subsystem
      settings: PortSchema="{\"entries\":[{\"content\":{\"headerSize\":26,\"margin\":15,\"minimumSpacing\":25,\"sides\":[{\"content\":{\"connectorIds\":[\"In1\"]},\"type\":\"ConnectorPlacement.EquallySpacedRectSide\",\"uuid\":\"2e13f5a1-d12d-4e78-8c7d-b3419191e00e\"},{\"content\":{\"side\":\"RIGHT\"},\"type\":\"ConnectorPlacement.EquallySpacedRectSide\",\"uuid\":\"2e54f79d-d26c-4f1e-aad7-d167a8605581\"},{\"content\":{\"side\":\"TOP\"},\"type\":\"ConnectorPlacement.EquallySpacedRectSide\",\"uuid\":\"127632d1-acf1-4856-b80a-47a4730bf8fe\"},{\"content\":{\"connectorIds\":[\"Out1\"],\"side\":\"BOTTOM\"},\"type\":\"ConnectorPlacement.EquallySpacedRectSide\",\"uuid\":\"4fc0a07c-a833-4ca9-b6fd-5fc8d4c0b5dc\"}]},\"type\":\"ConnectorPlacement.EquallySpacedConnector\",\"uuid\":\"7fb5950c-eb56-4ad7-bb81-f4b7b8097c7f\"}],\"packageUris\":[\"http://schema.mathworks.com/mf0/Connector/R2020b\"],\"version\":\"1.0\"}"
  Printed Circuit Board : Subsystem
      settings: PortSchema="{\"entries\":[{\"content\":{\"headerSize\":26,\"margin\":15,\"minimumSpacing\":25,\"sides\":[{\"content\":{},\"type\":\"ConnectorPlacement.EquallySpacedRectSide\",\"uuid\":\"2e13f5a1-d12d-4e78-8c7d-b3419191e00e\"},{\"content\":{\"connectorIds\":[\"Out1\",\"Out2\"],\"side\":\"RIGHT\"},\"type\":\"ConnectorPlacement.EquallySpacedRectSide\",\"uuid\":\"2e54f79d-d26c-4f1e-aad7-d167a8605581\"},{\"content\":{\"side\":\"TOP\"},\"type\":\"ConnectorPlacement.EquallySpacedRectSide\",\"uuid\":\"127632d1-acf1-4856-b80a-47a4730bf8fe\"},{\"content\":{\"connectorIds\":[\"In1\"],\"side\":\"BOTTOM\"},\"type\":\"ConnectorPlacement.EquallySpacedRectSide\",\"uuid\":\"84609f25-f9e8-4f57-ac2d-b4cbc4264e2d\"}]},\"type\":\"ConnectorPlacement.EquallySpacedConnector\",\"uuid\":\"7fb5950c-eb56-4ad7-bb81-f4b7b8097c7f\"}],\"packageUris\":[\"http://schema.mathworks.com/mf0/Connector/R2020b\"],\"version\":\"1.0\"}"
  Bus Element Out1 : Outport  PortName=Altitude Data
  Bus Element Out2 : Outport  Port=2  PortName=Data
  wires:
  Bus Element In1/1 -> Printed Circuit Board/1(Power)
  Printed Circuit Board/1(Altitude Data) -> Bus Element Out1/1
  Printed Circuit Board/2(Control Signals) -> Altimeter/1(Control Signals)
  Altimeter/1(Data) -> Bus Element Out2/1

== system LukePractice/Propulsion System/Igniter ==
  Bus Element In1 : Inport  PortName=Wire
  Bus Element In2 : Inport  Port=2  PortName=Ignition Signal
  Bus Element Out2 : Outport  PortName=OutBus
  Bus Element Out1 : Outport  Port=2  PortName=Spark

== system LukePractice/Propulsion System/Ignition System ==
  Bus Element In1 : Inport  PortName=Igniton Sequence
  Bus Element Out2 : Outport  PortName=Wired Connection
  Bus Element Out1 : Outport  Port=2  PortName=Ignition Signal
  Bus Element Out3 : Outport  Port=3  PortName=Wire

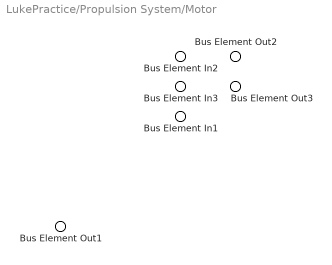
== system LukePractice/Propulsion System/Motor  ==
  Bus Element In1 : Inport  PortName=InBus
  Bus Element In3 : Inport  Port=2  PortName=Spark
  Bus Element In2 : Inport  Port=3  PortName=Wired Connection
  Bus Element Out3 : Outport  PortName=Bottom Mount
  Bus Element Out2 : Outport  Port=2  PortName=Top Mount
  Bus Element Out1 : Outport  Port=3  PortName=Thrust Force

== system LukePractice/Recovery System/Drogue Chute ==
  Bus Element In1 : Inport  PortName=Deployment Trigger
  Bus Element Out1 : Outport  PortName=OutBus

== system LukePractice/Recovery System/Main Chute ==
  Bus Element In1 : Inport  PortName=InBus
  Bus Element Out1 : Outport  PortName=Visible Chute

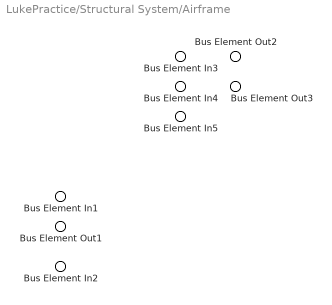
== system LukePractice/Structural System/Airframe ==
  Bus Element In3 : Inport  PortName=Stabilising Forces
  Bus Element In1 : Inport  Port=2  PortName=Force
  Bus Element In4 : Inport  Port=3  PortName=Physical Connection
  Bus Element In5 : Inport  Port=4  PortName=Coupler
  Bus Element In2 : Inport  Port=5  PortName=Body of Rocket
  Bus Element Out3 : Outport  PortName=OutBus
  Bus Element Out2 : Outport  Port=2  PortName=Acceleration/Orientation
  Bus Element Out1 : Outport  Port=3  PortName=Rigid Mount Positions for Fins

== system LukePractice/Structural System/Fins ==
  Bus Element In1 : Inport  PortName=Rigid Mount Positions for Fins
  X Fin : Subsystem
      settings: PortSchema="{\"entries\":[{\"content\":{\"headerSize\":26,\"margin\":15,\"minimumSpacing\":25,\"sides\":[{\"content\":{},\"type\":\"ConnectorPlacement.EquallySpacedRectSide\",\"uuid\":\"ee90fd67-ce3c-463a-922d-00379c91d92f\"},{\"content\":{\"connectorIds\":[\"Out1\"],\"side\":\"RIGHT\"},\"type\":\"ConnectorPlacement.EquallySpacedRectSide\",\"uuid\":\"57bdd80c-9026-4844-a97e-bdf46341acf9\"},{\"content\":{\"side\":\"TOP\"},\"type\":\"ConnectorPlacement.EquallySpacedRectSide\",\"uuid\":\"7c374427-6658-48c0-ad54-d8c414c813ef\"}]},\"type\":\"ConnectorPlacement.EquallySpacedConnector\",\"uuid\":\"baeb2d3f-30b1-4010-b9ee-d30a650b13c4\"}],\"packageUris\":[\"http://schema.mathworks.com/mf0/Connector/R2020b\"],\"version\":\"1.0\"}"
  Y Fin : Subsystem
      settings: PortSchema="{\"entries\":[{\"content\":{\"headerSize\":26,\"margin\":15,\"minimumSpacing\":25,\"sides\":[{\"content\":{\"connectorIds\":[\"In1\"]},\"type\":\"ConnectorPlacement.EquallySpacedRectSide\",\"uuid\":\"ee90fd67-ce3c-463a-922d-00379c91d92f\"},{\"content\":{\"side\":\"RIGHT\"},\"type\":\"ConnectorPlacement.EquallySpacedRectSide\",\"uuid\":\"57bdd80c-9026-4844-a97e-bdf46341acf9\"},{\"content\":{\"side\":\"TOP\"},\"type\":\"ConnectorPlacement.EquallySpacedRectSide\",\"uuid\":\"7c374427-6658-48c0-ad54-d8c414c813ef\"}]},\"type\":\"ConnectorPlacement.EquallySpacedConnector\",\"uuid\":\"baeb2d3f-30b1-4010-b9ee-d30a650b13c4\"}],\"packageUris\":[\"http://schema.mathworks.com/mf0/Connector/R2020b\"],\"version\":\"1.0\"}"
  Bus Element Out2 : Outport  PortName=Stabilising Forces
  Bus Element Out1 : Outport  Port=2  PortName=Control/Orientation
  wires:
  X Fin/1(OutBus) -> Y Fin/1(InBus)

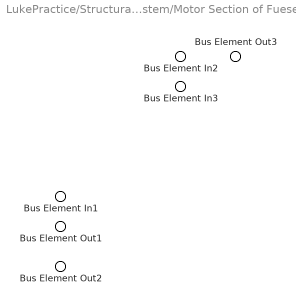
== system LukePractice/Structural System/Motor Section of Fueselage ==
  Bus Element In2 : Inport  PortName=Top Motor Mount
  Bus Element In3 : Inport  Port=2  PortName=Bottom Motor Mount
  Bus Element In1 : Inport  Port=3  PortName=Thrust Force
  Bus Element Out3 : Outport  PortName=Coupler
  Bus Element Out1 : Outport  Port=2  PortName=Force
  Bus Element Out2 : Outport  Port=3  PortName=Body of Rocket

== system LukePractice/Structural System/Payload Section of Fueselage ==
  Bus Element In1 : Inport  PortName=InBus
  Bus Element Out4 : Outport  PortName=Bolts for Launch Adapter
  Bus Element Out1 : Outport  Port=2  PortName=Physical Connection
  Bus Element Out3 : Outport  Port=3  PortName=Electricial Power
  Bus Element Out2 : Outport  Port=4  PortName=OutBus

== system LukePractice/Avionics System/Sensors/Altimeter ==
  Bus Element Out1 : Outport  PortName=Altitude Data

== system LukePractice/Avionics System/Sensors/Barometer ==
  Bus Element Out1 : Outport  PortName=Pressure Data

== system LukePractice/Payload System/Rideshare Payload/Altimeter ==
  Bus Element In1 : Inport  PortName=Control Signals
  Bus Element Out1 : Outport  PortName=Data

== system LukePractice/Payload System/Rideshare Payload/Printed Circuit Board ==
  Bus Element In1 : Inport  PortName=Power
  Bus Element Out1 : Outport  PortName=Altitude Data
  Bus Element Out2 : Outport  Port=2  PortName=Control Signals

== system LukePractice/Structural System/Fins/X Fin ==
  Bus Element Out1 : Outport  PortName=OutBus

== system LukePractice/Structural System/Fins/Y Fin ==
  Bus Element In1 : Inport  PortName=InBus
